simulink library "MPC_Sublibraries"  (R2020a)
settings: Solver=VariableStepAuto  StartTime=0.0  StopTime=10.0  RelTol=1e-3
(part 2 of 2)

== matlab function MPC_Sublibraries/Pre-MPC v0 ==
  data: States input size=4; Scalar_Out output; Env output size=51; Param input; Route input; T_p input; V_new input; KE_des output size=51; KE_max output size=51; KE_min output size=51; lam_b output size=51; lam_e output size=51; V_des_0 output; dx input
function [Scalar_Out,Env,KE_des,KE_max,KE_min,lam_b,lam_e,V_des_0] = ...
    fcn(States,Param,Route,T_p,V_new,dx)
%%  Extract Inputs
t_0 = States(3);                                        %   s - Sim time
x_0 = States(1);                                        %   m - Current position
v_0 = States(2);                                        %   m/s - Current velocity 
GR = States(4);                                         %   Current Gear
g = Param(1);                                           %   m/s^2 - Accel due to gravity
rho = Param(2);                                         %   kg/m^3 - Air density
m = Param(3);                                           %   kg - Base vehicle mass
Cd = Param(4);                                          %   Drag Coefficient
A_ref = Param(5);                                       %   m^2 - Reference area
Cr = Param(6);                                          %   Rolling resistance coefficient
r_wh = Param(7);                                        %   m - Wheel radius
X_vec = Route(:,1);                                     %   rad - Road grade angle vector
theta_vec = Route(:,2);                                 %   rad - Road grade angle vector
V_lim = Route(:,3);                                     %   m/s - Current speed limit
%%  Controller Setup
dx = 10;                                                %   m - Position step
NP = 51;                                                %   # of pred steps
x_pred = x_0+dx*NP-dx;                                  %   m - Prediction horizon length
XP = (linspace(x_0,x_pred,NP))';                        %   m - Position vector
%%  Horizon Vectors
V_des = V_new*ones(numel(XP),1);                                    %   m/s - Initialize des velocty vector
v_lim = interp1(X_vec,V_lim,XP,'previous',V_lim(end));              %   m/s - Maximum velocity vector 
v_min = 0*v_lim;                                                    %   m/s - Minimum velocity vector 
theta = interp1(X_vec,theta_vec,XP,'linear',theta_vec(end));        %   rad - Road grade vector 
KE_max = .5*m*v_lim.^2;                                             %   J - Maximum kinetic energy vector 
KE_min = .5*m*v_min.^2;                                             %   J - Minimum kinetic energy vector 
F_grav = m*g*sin(theta);                                            %   N - Gravitational force vector 
F_road = m*g*Cr*cos(theta);                                         %   N - Rolling resistance force vector 
Env = (F_road+F_grav)*dx;                                           %   J - Environmental resistance energy vector 
%%  Prepare MPC parameters
V_des_0 = V_des(1);                                     %   m/s - 1st desired velocity 
A = 1-1/m*rho*Cd*A_ref*dx;                              %   Dynamics matrix
KE_0 = 1/2*m*v_0^2;                                     %   J - Initial kinetic energy 
F_wh_max = min(2200.*2.47*GR/r_wh,80000);               %   N - Maximum control force
E_mech_max = F_wh_max*dx;                               %   J - Initial max ME
E_mech_min = 0;                                         %   J - Mechanical energy lower limit 
E_brk_max = 35000*dx;                                   %   J - Brake energy upper limit 
E_brk_min = 0;                                          %   J - Brake energy lower limit 
U_p = T_p/r_wh*dx;                                      %   Previous control value
dU = 1e5;                                               %   J - Max control step
KE_des = 1/2*m.*V_des.^2;                               %   J - Initialize desired KE vector
if dx > 250
    lam_e = 1e1*ones(NP,1); lam_b = 1e3*ones(NP,1);
elseif dx <= 250
    lam_e = 1e3*ones(NP,1); lam_b = 1e-1*ones(NP,1);
end

Scalar_Out = [A,KE_0,E_mech_max,E_mech_min,...
    E_brk_max,E_brk_min,U_p,dU]';
